simulink model "RIPNS_v01_R2015a"  (R2015b)
settings: Solver=ode45  StartTime=0.0  StopTime=tfinal  FixedStep=0.005  RelTol=1e-3
values from neighbouring files (symbols this model uses):
  A = [ 0         0    1.0000         0 ... (first row only)    [ROTPEN_Sim_Setup.m]
  B = [     0 ... (first row only)    [ROTPEN_Sim_Setup.m]
  C = [eye(2),zeros(2,2)]    [ROTPEN_Sim_Setup.m]
  control_threshold = 12*pi/180    (= 0.209439510239)    [ROTPEN_Sim_Setup.m]
  D = zeros(2,1)    [ROTPEN_Sim_Setup.m]
  eta_g = 9.0000*10^-1    (= 0.9)    [ROTPEN_Sim_Setup.m]
  eta_m = 6.899999999999999*10^-1    (= 0.69)    [ROTPEN_Sim_Setup.m]
  IC = [0,0,0,0]*pi/180.'    [ROTPEN_Sim_Setup.m]
  K = [-8.5311, 45.7674, -4.1375, 5.2391]    [ROTPEN_Sim_Setup.m]
  Kg = 70    [ROTPEN_Sim_Setup.m]
  km = 7.677634454753032*10^-3    (= 0.00767763445475)    [ROTPEN_Sim_Setup.m]
  kt = 7.682969729279999*10^-3    (= 0.00768296972928)    [ROTPEN_Sim_Setup.m]
  Parameters = [Mp,Lr,Lp,Jr,Jp,Br,Bp,g].'    [ROTPEN_Sim_Setup.m]
  Rm = 2.6000    (= 2.6)    [ROTPEN_Sim_Setup.m]
  slew_fall = -inf*pi/180    (= -inf)    [ROTPEN_Sim_Setup.m]
  slew_rise = inf*pi/180    (= inf)    [ROTPEN_Sim_Setup.m]
  square_amp = 10*pi/180    (= 0.174532925199)    [ROTPEN_Sim_Setup.m]
  square_freq = 1/5    (= 0.2)    [ROTPEN_Sim_Setup.m]
  wcf_1 = 62.831853071795862    (= 62.8318530718)    [ROTPEN_Sim_Setup.m]
  wcf_2 = wcf_1    (= 62.8318530718)    [ROTPEN_Sim_Setup.m]
Description:
  | Rotary Inverted Pendulum Nonlinear Simulation
  | D. Hartman, 1/20/16
settings Model: Creator=davidhartman  LastModifiedBy=davidhartman
settings SolverCC: MaxConsecutiveMinStep=100  ShapePreserveControl=EnableAll  ZeroCrossControl=DisableAll
settings DataIOCC: LimitDataPoints=off
settings HardwareCC: ProdWordSize=32  ProdHWDeviceType=Specified

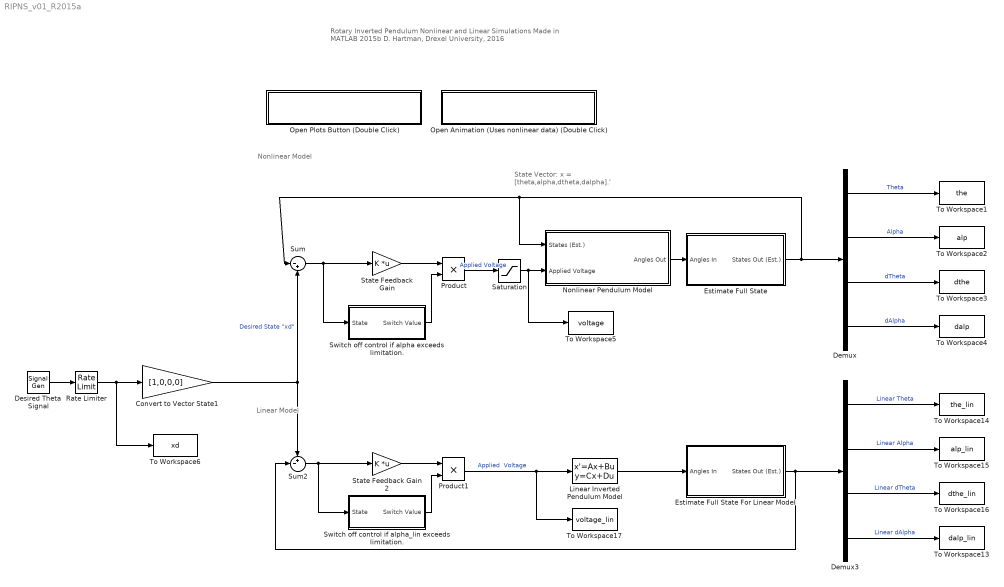
== system RIPNS_v01_R2015a ==
  note: Linear Model
  note: Nonlinear Model
  note: Rotary Inverted Pendulum
      | Nonlinear and Linear Simulations
      | Made in MATLAB 2015b
      | D. Hartman, Drexel University, 2016
  note: State Vector:
      | x = [theta,alpha,dtheta,dalpha].'
  Convert to Vector State1 : Gain  Gain=[1,0,0,0]
  Demux : Demux
  Demux3 : Demux
  Desired Theta Signal : SignalGenerator  WaveForm=square  Amplitude=square_amp  Frequency=square_freq
  Estimate Full State : Subsystem
  Estimate Full State For Linear Model : Subsystem
  Linear Inverted Pendulum Model : StateSpace  A=A  B=B  C=C  D=D  X0=IC
  Nonlinear Pendulum Model : Subsystem
  Open Animation (Uses nonlinear data) (Double Click) : Subsystem
      settings: OpenFcn=RIPNS_Animation_v01(the, alp, the_lin, alp_lin, control_threshold, tout)
      mask Display: fprintf('OPEN ANIMATION')
  Open Plots Button (Double Click) : Subsystem
      settings: OpenFcn=RIPNS_Plot_v01(the,alp,dthe,dalp,voltage,the_lin,alp_lin,dthe_lin,dalp_lin,voltage_lin,xd,tout)
      mask Display: fprintf('OPEN PLOT: State Data')
  Product : Product  OutDataTypeStr=Inherit: Same as first input
  Product1 : Product  OutDataTypeStr=Inherit: Same as first input
  Rate Limiter : RateLimiter  RisingSlewLimit=slew_rise  FallingSlewLimit=slew_fall  SampleTimeMode=inherited
  Saturation : Saturate  UpperLimit=5  LowerLimit=-5
  State Feedback Gain : Gain  Gain=K  Multiplication=Matrix(K*u)
  State Feedback Gain 2 : Gain  Gain=K  Multiplication=Matrix(K*u)
  Sum : Sum  Inputs=|-+
  Sum2 : Sum  Inputs=+-|
  Switch off control if alpha exceeds limitation. : Subsystem
  Switch off control if alpha_lin exceeds limitation. : Subsystem
  To Workspace1 : ToWorkspace  VariableName=the  SampleTime=-1
      settings: Save2DSignal=2-D array (concatenate along first dimension)
  To Workspace13 : ToWorkspace  VariableName=dalp_lin  SampleTime=-1
      settings: Save2DSignal=2-D array (concatenate along first dimension)
  To Workspace14 : ToWorkspace  VariableName=the_lin  SampleTime=-1
      settings: Save2DSignal=2-D array (concatenate along first dimension)
  To Workspace15 : ToWorkspace  VariableName=alp_lin  SampleTime=-1
      settings: Save2DSignal=2-D array (concatenate along first dimension)
  To Workspace16 : ToWorkspace  VariableName=dthe_lin  SampleTime=-1
      settings: Save2DSignal=2-D array (concatenate along first dimension)
  To Workspace17 : ToWorkspace  VariableName=voltage_lin  SampleTime=-1
      settings: Save2DSignal=2-D array (concatenate along first dimension)
  To Workspace2 : ToWorkspace  VariableName=alp  SampleTime=-1
      settings: Save2DSignal=2-D array (concatenate along first dimension)
  To Workspace3 : ToWorkspace  VariableName=dthe  SampleTime=-1
      settings: Save2DSignal=2-D array (concatenate along first dimension)
  To Workspace4 : ToWorkspace  VariableName=dalp  SampleTime=-1
      settings: Save2DSignal=2-D array (concatenate along first dimension)
  To Workspace5 : ToWorkspace  VariableName=voltage  SampleTime=-1
      settings: Save2DSignal=2-D array (concatenate along first dimension)
  To Workspace6 : ToWorkspace  VariableName=xd  SampleTime=-1
      settings: Save2DSignal=2-D array (concatenate along first dimension)
  wires:
  Demux/4 -> To Workspace4/1  "dAlpha"
  Demux/3 -> To Workspace3/1  "dTheta"
  Demux/2 -> To Workspace2/1  "Alpha"
  Demux/1 -> To Workspace1/1  "Theta"
  Sum/1 -> State Feedback Gain/1, Switch off control if alpha exceeds limitation./1(State)
  Switch off control if alpha exceeds limitation./1(Switch Value) -> Product/2
  State Feedback Gain/1 -> Product/1
  Desired Theta Signal/1 -> Rate Limiter/1
  Rate Limiter/1 -> To Workspace6/1, Convert to Vector State1/1
  Convert to Vector State1/1 -> Sum/2, Sum2/1  "Desired State \"xd\""
  Sum2/1 -> State Feedback Gain 2/1, Switch off control if alpha_lin exceeds limitation./1(State)
  Estimate Full State For Linear Model/1(States Out (Est.)) -> Sum2/2, Demux3/1
  Demux3/1 -> To Workspace14/1  "Linear Theta"
  Demux3/2 -> To Workspace15/1  "Linear Alpha"
  Demux3/3 -> To Workspace16/1  "Linear dTheta"
  Demux3/4 -> To Workspace13/1  "Linear dAlpha"
  Nonlinear Pendulum Model/1(Angles Out) -> Estimate Full State/1(Angles In)
  Estimate Full State/1(States Out (Est.)) -> Demux/1, Nonlinear Pendulum Model/1(States (Est.)), Sum/1
  Linear Inverted Pendulum Model/1 -> Estimate Full State For Linear Model/1(Angles In)
  Product1/1 -> Linear Inverted Pendulum Model/1, To Workspace17/1  "Applied  Voltage"
  State Feedback Gain 2/1 -> Product1/1
  Switch off control if alpha_lin exceeds limitation./1(Switch Value) -> Product1/2
  Product/1 -> Saturation/1  "Applied Voltage"
  Saturation/1 -> To Workspace5/1, Nonlinear Pendulum Model/2(Applied Voltage)

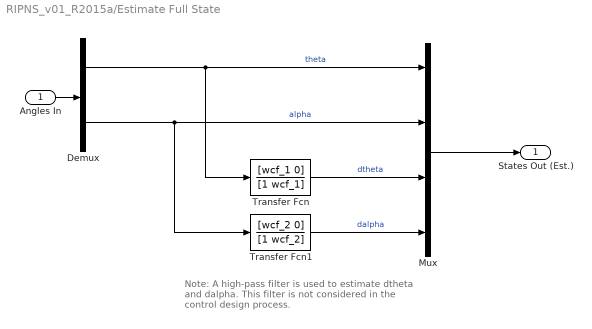
== system RIPNS_v01_R2015a/Estimate Full State ==
  note: Note: A high-pass filter is used to estimate
      | dtheta and dalpha. This filter is not considered
      | in the control design process.
  Angles In : Inport
  Demux : Demux  Outputs=2
  Mux : Mux
  Transfer Fcn : TransferFcn  Numerator=[wcf_1 0]  Denominator=[1 wcf_1]
  Transfer Fcn1 : TransferFcn  Numerator=[wcf_2 0]  Denominator=[1 wcf_2]
  States Out (Est.) : Outport
  wires:
  Transfer Fcn1/1 -> Mux/4  "dalpha"
  Mux/1 -> States Out (Est.)/1
  Transfer Fcn/1 -> Mux/3  "dtheta"
  Angles In/1 -> Demux/1
  Demux/1 -> Transfer Fcn/1, Mux/1  "theta"
  Demux/2 -> Transfer Fcn1/1, Mux/2  "alpha"

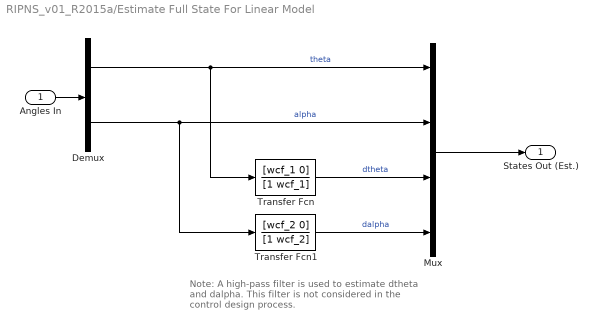
== system RIPNS_v01_R2015a/Estimate Full State For Linear Model ==
  note: Note: A high-pass filter is used to estimate
      | dtheta and dalpha. This filter is not considered
      | in the control design process.
  Angles In : Inport
  Demux : Demux  Outputs=2
  Mux : Mux
  Transfer Fcn : TransferFcn  Numerator=[wcf_1 0]  Denominator=[1 wcf_1]
  Transfer Fcn1 : TransferFcn  Numerator=[wcf_2 0]  Denominator=[1 wcf_2]
  States Out (Est.) : Outport
  wires:
  Transfer Fcn1/1 -> Mux/4  "dalpha"
  Mux/1 -> States Out (Est.)/1
  Transfer Fcn/1 -> Mux/3  "dtheta"
  Angles In/1 -> Demux/1
  Demux/1 -> Transfer Fcn/1, Mux/1  "theta"
  Demux/2 -> Transfer Fcn1/1, Mux/2  "alpha"

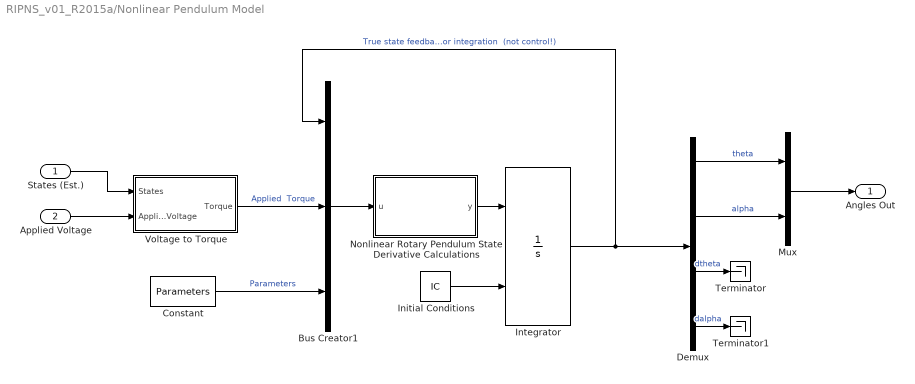
== system RIPNS_v01_R2015a/Nonlinear Pendulum Model ==
  States (Est.) : Inport
  Applied Voltage : Inport  Port=2
  Bus Creator1 : BusCreator  Inputs=3
  Constant : Constant  Value=Parameters
  Demux : Demux
  Initial Conditions : Constant  Value=IC
  Integrator : Integrator  InitialConditionSource=external
  Mux : Mux  Inputs=2
  Nonlinear Rotary Pendulum State Derivative Calculations : MATLAB Function  TreatAsAtomicUnit=on
  Terminator : Terminator
  Terminator1 : Terminator
  Voltage to Torque : Subsystem
  Angles Out : Outport
  wires:
  States (Est.)/1 -> Voltage to Torque/1(States)
  Nonlinear Rotary Pendulum State Derivative Calculations/1(y) -> Integrator/1
  Bus Creator1/1 -> Nonlinear Rotary Pendulum State Derivative Calculations/1(u)
  Constant/1 -> Bus Creator1/3  "Parameters"
  Integrator/1 -> Demux/1, Bus Creator1/1  "True state feedback for integration  (not control!)"
  Initial Conditions/1 -> Integrator/2
  Applied Voltage/1 -> Voltage to Torque/2(Applied Voltage)
  Voltage to Torque/1(Torque) -> Bus Creator1/2  "Applied  Torque"
  Demux/3 -> Terminator/1  "dtheta"
  Demux/4 -> Terminator1/1  "dalpha"
  Demux/1 -> Mux/1  "theta"
  Demux/2 -> Mux/2  "alpha"
  Mux/1 -> Angles Out/1

== system RIPNS_v01_R2015a/Open Animation (Uses nonlinear data) (Double Click) ==

== system RIPNS_v01_R2015a/Open Plots Button (Double Click) ==

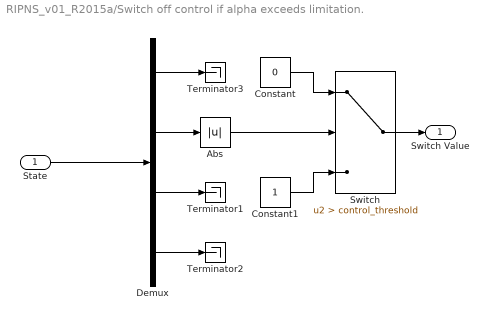
== system RIPNS_v01_R2015a/Switch off control if alpha exceeds limitation. ==
  State : Inport
  Abs : Abs
  Constant : Constant  Value=0
  Constant1 : Constant
  Demux : Demux
  Switch : Switch  Criteria=u2 > Threshold  Threshold=control_threshold  ZeroCross=off
  Terminator1 : Terminator
  Terminator2 : Terminator
  Terminator3 : Terminator
  Switch Value : Outport  PortDimensions=1
  wires:
  State/1 -> Demux/1
  Demux/2 -> Abs/1
  Demux/3 -> Terminator1/1
  Demux/4 -> Terminator2/1
  Constant/1 -> Switch/1
  Constant1/1 -> Switch/3
  Switch/1 -> Switch Value/1
  Demux/1 -> Terminator3/1
  Abs/1 -> Switch/2

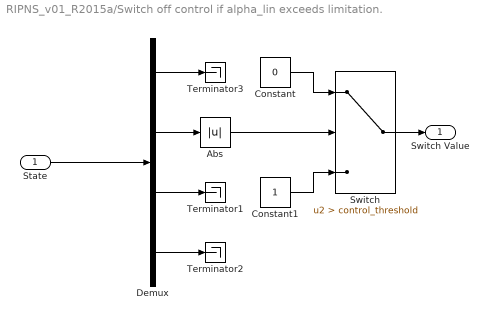
== system RIPNS_v01_R2015a/Switch off control if alpha_lin exceeds limitation. ==
  State : Inport
  Abs : Abs
  Constant : Constant  Value=0
  Constant1 : Constant
  Demux : Demux
  Switch : Switch  Criteria=u2 > Threshold  Threshold=control_threshold  ZeroCross=off
  Terminator1 : Terminator
  Terminator2 : Terminator
  Terminator3 : Terminator
  Switch Value : Outport  PortDimensions=1
  wires:
  State/1 -> Demux/1
  Demux/2 -> Abs/1
  Demux/3 -> Terminator1/1
  Demux/4 -> Terminator2/1
  Constant/1 -> Switch/1
  Constant1/1 -> Switch/3
  Switch/1 -> Switch Value/1
  Demux/1 -> Terminator3/1
  Abs/1 -> Switch/2

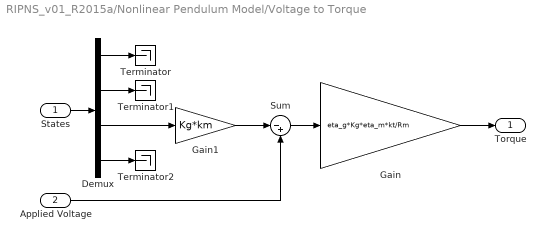
== system RIPNS_v01_R2015a/Nonlinear Pendulum Model/Voltage to Torque ==
  States : Inport
  Applied Voltage : Inport  Port=2
  Demux : Demux
  Gain : Gain  Gain=eta_g*Kg*eta_m*kt/Rm
  Gain1 : Gain  Gain=Kg*km
  Sum : Sum  Inputs=|-+
  Terminator : Terminator
  Terminator1 : Terminator
  Terminator2 : Terminator
  Torque : Outport  PortDimensions=1
  wires:
  Gain/1 -> Torque/1
  Applied Voltage/1 -> Sum/2
  States/1 -> Demux/1
  Sum/1 -> Gain/1
  Demux/3 -> Gain1/1
  Demux/1 -> Terminator/1
  Demux/2 -> Terminator1/1
  Demux/4 -> Terminator2/1
  Gain1/1 -> Sum/1

== matlab function RIPNS_v01_R2015a/Nonlinear Pendulum Model/Nonlinear Rotary Pendulum State Derivative Calculations ==
  data: u input; y output
function y = fcn(u)
%#codegen
% Simulink "MATLAB function block" code to calculate state derivatives
% for Rotary Inverted Pendulum Nonlinear Simulation
% D. Hartman

% Extract State Variables and Parameters From Input 
x1 = u(1); x2 = u(2); x3 = u(3); x4 = u(4); tau = u(5);
% parameters order: [Mp,Lr,Lp,Jr,Jp,Br,Bp,g].';
Mp  = u(6); Lr = u(7); Lp = u(8); Jr = u(9); Jp = u(10); 
Br = u(11); Bp = u(12); g = u(13);

% Calculate dx1:
dx1 = x3;

% Calculate dx2:
dx2 = x4;

% Calculate dx4:
dx4 = (2*Lp*Mp*(8*Lr*tau*cos(x2) + ...
      g*(8*Jr + Lp^2*Mp + 8*Lr^2*Mp - Lp^2*Mp*cos(2*x2))*sin(x2)) + ...
   1/2*Lp^2*Mp*(8*Jr + Lp^2*Mp + 8*Lr^2*Mp - ... 
      Lp^2*Mp*cos(2*x2))*sin(2*x2)*x3^2 - ...
   4*Lp*Lr*Mp*cos(x2)*x3*(4*Br + Lp^2*Mp*sin(2*x2)*x4) - ... 
   4*x4*(Bp*(8*Jr + Lp^2*Mp + 8*Lr^2*Mp - Lp^2*Mp*cos(2*x2)) + ... 
      Lp^2*Lr^2*Mp^2*sin(2*x2)*x4))/(-8*Lp^2*Lr^2*Mp^2*cos(x2)^2 + ...
      (4*Jp + Lp^2*Mp)*(8*Jr + Lp^2*Mp + 8*Lr^2*Mp - ...
      Lp^2*Mp*cos(2*x2)));

% Calculate dx3 (note dependance on dx4! Could be eliminated via 
% substitution of course, but that makes the code longer.):
dx3 = (8*tau - 2*x3*(4*Br + Lp^2*Mp*sin(2*x2)*x4) + ...
   4*Lp*Lr*Mp*(-sin(x2)*x4^2 + ...
      cos(x2)*dx4))/(8*Jr + (Lp^2 + 8*Lr^2)*Mp - ...
   Lp^2*Mp*cos(2*x2));

% Form output vector y, containing all of the state derivatives:
y = [dx1, dx2, dx3, dx4].';
